simulink model "admire_fcs_lin_incl_cs"  (Simulink 3.00)
settings: Solver=ode4  SolverMode=SingleTasking  StartTime=0.0  StopTime=60  FixedStep=0.008  RelTol=1e-3  AbsTol=1e-6
values from neighbouring files (symbols this model uses):
  x0 = [ max(eyp,zeros(n,1));max(-eyp,zeros(n,1));zeros(2*m,1)]    [LPwrap.m]
undefined symbols (not defined in the file or in its folder): Alt, dalt_err, dMach_err, Mach, u0fcs, y0bare
libraries: simulink3 x22, simulink_extras x8
(part 2 of 2)

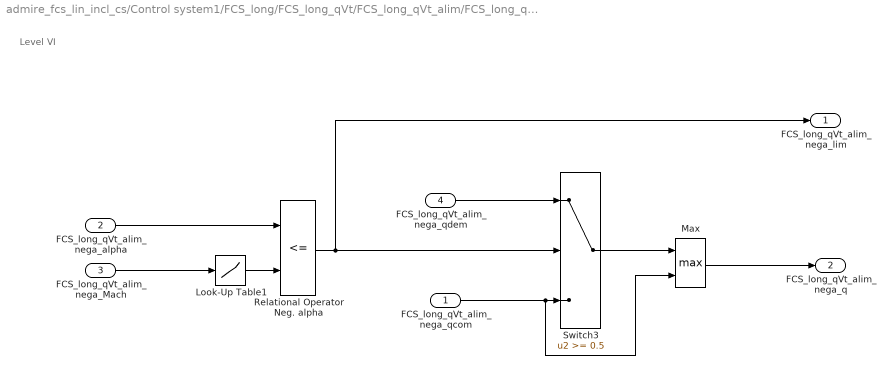
== system admire_fcs_lin_incl_cs/Control system1/FCS_long/FCS_long_qVt/FCS_long_qVt_alim/FCS_long_qVt_alim_nega ==
  note: Level VI
  "FCS_long_qVt_alim_nega_qcom " : Inport  Port=1  PortWidth=-1  SampleTime=-1  DataType=auto
      settings: SignalType=auto
  "FCS_long_qVt_alim_nega_alpha " : Inport  Port=2  PortWidth=-1  SampleTime=-1  DataType=auto
      settings: SignalType=auto
  "FCS_long_qVt_alim_nega_Mach " : Inport  Port=3  PortWidth=-1  SampleTime=-1  DataType=auto
      settings: SignalType=auto
  "FCS_long_qVt_alim_nega_qdem " : Inport  Port=4  PortWidth=-1  SampleTime=-1  DataType=auto
      settings: SignalType=auto
  Look-Up Table1 : Lookup  InputValues=[0 1 1 2.5]  OutputValues=[-8 -8 -3 -3]
  Max : MinMax  Function=max  Inputs=2
  Relational Operator Neg. alpha : RelationalOperator  Operator=<=
  Switch3 : Switch  Threshold=0.5
  FCS_long_qVt_alim_nega_lim : Outport  Port=1
  "FCS_long_qVt_alim_nega_q " : Outport  Port=2
  wires:
  "FCS_long_qVt_alim_nega_Mach "/1 -> Look-Up Table1/1
  Look-Up Table1/1 -> Relational Operator Neg. alpha/2
  "FCS_long_qVt_alim_nega_alpha "/1 -> Relational Operator Neg. alpha/1
  Max/1 -> "FCS_long_qVt_alim_nega_q "/1
  "FCS_long_qVt_alim_nega_qdem "/1 -> Switch3/1
  Relational Operator Neg. alpha/1 -> Switch3/2, FCS_long_qVt_alim_nega_lim/1
  Switch3/1 -> Max/1
  "FCS_long_qVt_alim_nega_qcom "/1 -> Switch3/3, Max/2

== system admire_fcs_lin_incl_cs/Control system1/FCS_long/FCS_long_qVt/FCS_long_qVt_alim/FCS_long_qVt_alim_posa ==
  note: Level VI
  "FCS_long_qVt_alim_posa_qcom " : Inport  Port=1  PortWidth=-1  SampleTime=-1  DataType=auto
      settings: SignalType=auto
  "FCS_long_qVt_alim_posa_alpha " : Inport  Port=2  PortWidth=-1  SampleTime=-1  DataType=auto
      settings: SignalType=auto
  "FCS_long_qVt_alim_posa_Mach " : Inport  Port=3  PortWidth=-1  SampleTime=-1  DataType=auto
      settings: SignalType=auto
  "FCS_long_qVt_alim_posa_qdem " : Inport  Port=4  PortWidth=-1  SampleTime=-1  DataType=auto
      settings: SignalType=auto
  Look-Up Table : Lookup  InputValues=[0 0.8 0.8 1 1 1.3 1.3 2.5 ]  OutputValues=[28 28 23 23 18 18 13 13 ]
  Min : MinMax  Function=min  Inputs=2
  Relational Operator Pos. alpha : RelationalOperator  Operator=>=
  Switch2 : Switch  Threshold=0.5
  FCS_long_qVt_alim_posa_q : Outport  Port=1
  FCS_long_qVt_alim_posa_lim : Outport  Port=2
  wires:
  "FCS_long_qVt_alim_posa_alpha "/1 -> Relational Operator Pos. alpha/1
  "FCS_long_qVt_alim_posa_Mach "/1 -> Look-Up Table/1
  Look-Up Table/1 -> Relational Operator Pos. alpha/2
  Relational Operator Pos. alpha/1 -> Switch2/2, FCS_long_qVt_alim_posa_lim/1
  "FCS_long_qVt_alim_posa_qdem "/1 -> Switch2/1
  Min/1 -> FCS_long_qVt_alim_posa_q/1
  Switch2/1 -> Min/1
  "FCS_long_qVt_alim_posa_qcom "/1 -> Switch2/3, Min/2
